simulink model "sampleModel1662"  (R2023a)
settings: Solver=VariableStepAuto  StartTime=0.0  StopTime=10.0  RelTol=1e-3
libraries: hdlsllib x5, simulink x2
settings Model: Creator=user1  LastModifiedBy=user1

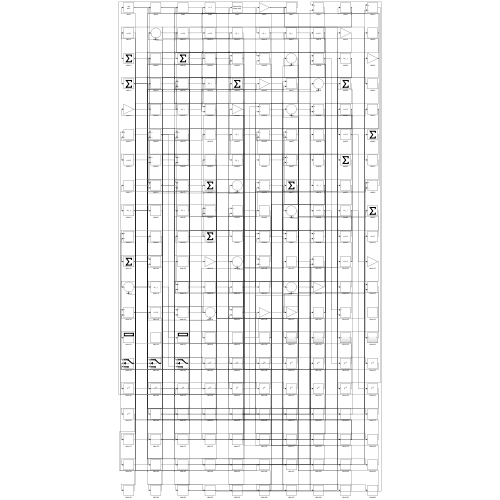
[thumbnail: Simulink's stored preview of the top-level diagram]
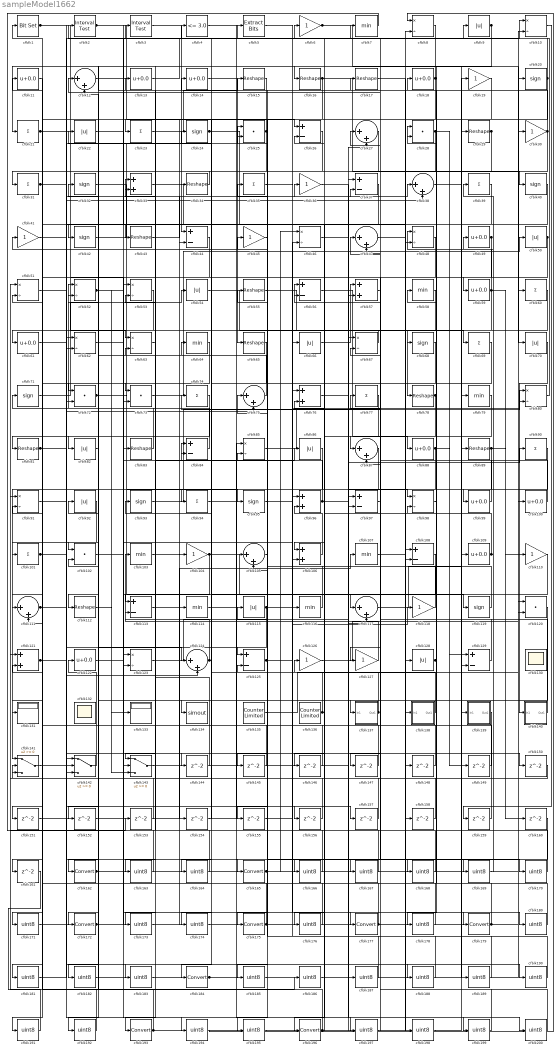
== system sampleModel1662 ==
  cfblk1 : simulink/Logic and Bit Operations/Bit Set  iBit=0
      settings: LibrarySourceBlock=|
      | hdlsllib/Logic and Bit
      | Operations/Bit Set
  cfblk{8,10,46,48,51..53,62..63,67,80,85,91,98,123} (15 alike) : Product  Inputs=*/  RndMeth=Zero  SaturateOnIntegerOverflow=on
  cfblk{11,13..14,18,49,59,61,88,99..100,109,122} (12 alike) : Bias  Bias=0.0  SaturateOnIntegerOverflow=off
  cfblk{21,23,31,35,39,60,69,74,77,90,94,101} (12 alike) : Sum  Inputs=+
  cfblk{25,28,72..73,102,120} (6 alike) : DotProduct  OutDataTypeStr=Inherit: Inherit via internal rule
  cfblk{7,58,64,79,103,107,114,116} (8 alike) : MinMax
  cfblk{6,19,30,36,41,45,104,110,118,126..127} (11 alike) : Gain
  cfblk{12,27,38,47,75,87,105,111,117,124} (10 alike) : Sum  Inputs=|++
  cfblk{33,57,76,96,106,121} (6 alike) : Sum
  cfblk{26,37,44,56,84,97,108,113,125,129} (10 alike) : Sum  Inputs=+-
  cfblk{15..17,29,34,43,55,65,78,81,83,89,112} (13 alike) : Reshape
  cfblk{9,22,50,54,66,70,82,86,92,115,128} (11 alike) : Abs  SaturateOnIntegerOverflow=off
  cfblk{20,24,32,40,42,68,71,93,95,119} (10 alike) : Signum
  cfblk130 : Scope
      settings: Floating=on
  cfblk131 : Display
  cfblk132 : Scope
      settings: Floating=on
  cfblk133 : Display
  cfblk134 : ToWorkspace  VariableName=simout  SaveFormat=Timeseries  SampleTime=-1
  cfblk135 : hdlsllib/Sources/Counter Limited  uplimit=7  tsamp=-1
  cfblk136 : hdlsllib/Sources/Counter Limited  uplimit=7  tsamp=-1
  cfblk137 : Subsystem
      settings: LibrarySourceBlock=|
      | hdlsllib/Ports &
      | Subsystems/Subsystem
  cfblk138 : Subsystem
      settings: LibrarySourceBlock=|
      | hdlsllib/Ports &
      | Subsystems/Subsystem
  cfblk139 : Subsystem
      settings: LibrarySourceBlock=|
      | hdlsllib/Ports &
      | Subsystems/Subsystem
  cfblk140 : Subsystem
      settings: LibrarySourceBlock=|
      | hdlsllib/Ports &
      | Subsystems/Subsystem
  cfblk141 : Switch  SaturateOnIntegerOverflow=off  InputSameDT=off
  cfblk142 : Switch  SaturateOnIntegerOverflow=off  InputSameDT=off
  cfblk143 : Switch  SaturateOnIntegerOverflow=off  InputSameDT=off
  cfblk{144..161} (18 alike) : Delay  SampleTime=1
  cfblk{162,165,172,175,177,179,184,193,196} (9 alike) : DataTypeConversion  SaturateOnIntegerOverflow=off  RndMeth=Floor
  cfblk{163..164,166..171,173..174,176,178,180..183,185..192,194..195,197..200} (30 alike) : DataTypeConversion  OutDataTypeStr=uint8  SaturateOnIntegerOverflow=off  RndMeth=Floor
  cfblk2 : hdlsllib/Logic and Bit Operations/Interval Test  IntervalClosedRight=on  uplimit=0.5  IntervalClosedLeft=on  lowlimit=-0.5  OutDataTypeStr=boolean
  cfblk3 : hdlsllib/Logic and Bit Operations/Interval Test  IntervalClosedRight=on  uplimit=0.5  IntervalClosedLeft=on  lowlimit=-0.5  OutDataTypeStr=boolean
  cfblk4 : hdlsllib/Logic and Bit Operations/Compare To Constant  relop=<=  const=3.0  OutDataTypeStr=boolean
  cfblk5 : simulink/Logic and Bit Operations/Extract Bits  bitsToExtract=Upper half  numBits=8  bitIdxRange=[0 7]  outScalingMode=Preserve fixed-point scaling
      settings: LibrarySourceBlock=|
      | hdlsllib/Logic and Bit
      | Operations/Extract Bits
  wires:
  cfblk31/1 -> cfblk10/1, cfblk43/1, cfblk166/1
  cfblk70/1 -> cfblk140/1(In1)
  cfblk80/1 -> cfblk9/1
  cfblk108/1 -> cfblk184/1
  cfblk50/1 -> cfblk101/1, cfblk155/1
  cfblk45/1 -> cfblk175/1
  cfblk56/1 -> cfblk88/1
  cfblk49/1 -> cfblk59/1, cfblk173/1
  cfblk93/1 -> cfblk80/1
  cfblk32/1 -> cfblk117/1
  cfblk30/1 -> cfblk21/1, cfblk72/2
  cfblk126/1 -> cfblk30/1
  cfblk14/1 -> cfblk65/1
  cfblk123/1 -> cfblk90/1
  cfblk51/1 -> cfblk165/1
  cfblk115/1 -> cfblk66/1, cfblk192/1
  cfblk90/1 -> cfblk106/1
  cfblk23/1 -> cfblk15/1
  cfblk127/1 -> cfblk103/1
  cfblk68/1 -> cfblk134/1
  cfblk121/1 -> cfblk75/2, cfblk183/1
  cfblk67/1 -> cfblk61/1
  cfblk1/1 -> cfblk63/1, cfblk124/2
  cfblk138/1(Out1) -> cfblk84/1
  cfblk73/1 -> cfblk50/1
  cfblk87/1 -> cfblk141/1
  cfblk72/1 -> cfblk95/1, cfblk7/1
  cfblk34/1 -> cfblk31/1
  cfblk104/1 -> cfblk119/1, cfblk143/2
  cfblk59/1 -> cfblk87/1, cfblk48/1, cfblk110/1
  cfblk5/1 -> cfblk116/1
  cfblk71/1 -> cfblk54/1
  cfblk95/1 -> cfblk80/2
  cfblk58/1 -> cfblk78/1
  cfblk44/1 -> cfblk102/1
  cfblk98/1 -> cfblk58/1
  cfblk83/1 -> cfblk52/1
  cfblk36/1 -> cfblk97/1
  cfblk18/1 -> cfblk16/1, cfblk73/1, cfblk42/1
  cfblk112/1 -> cfblk133/1
  cfblk28/1 -> cfblk149/1, cfblk163/1
  cfblk97/1 -> cfblk127/1
  cfblk66/1 -> cfblk57/1
  cfblk117/1 -> cfblk89/1
  cfblk25/1 -> cfblk23/1, cfblk72/1
  cfblk16/1 -> cfblk40/1, cfblk142/3
  cfblk128/1 -> cfblk28/1, cfblk98/2
  cfblk143/1 -> cfblk67/1
  cfblk100/1 -> cfblk56/1
  cfblk65/1 -> cfblk94/1
  cfblk53/1 -> cfblk162/1
  cfblk81/1 -> cfblk37/2, cfblk38/1, cfblk169/1
  cfblk139/1(Out1) -> cfblk141/2
  cfblk142/1 -> cfblk122/1
  cfblk74/1 -> cfblk131/1
  cfblk12/1 -> cfblk104/1
  cfblk77/1 -> cfblk196/1
  cfblk21/1 -> cfblk83/1, cfblk111/1
  cfblk55/1 -> cfblk69/1
  cfblk42/1 -> cfblk25/1
  cfblk136/1 -> cfblk22/1, cfblk6/1
  cfblk3/1 -> cfblk44/1
  cfblk89/1 -> cfblk99/1, cfblk113/1, cfblk160/1
  cfblk119/1 -> cfblk41/1
  cfblk9/1 -> cfblk68/1, cfblk152/1
  cfblk20/1 -> cfblk2/1, cfblk34/1
  cfblk85/1 -> cfblk19/1
  cfblk2/1 -> cfblk26/1, cfblk48/2
  cfblk135/1 -> cfblk20/1
  cfblk118/1 -> cfblk27/1
  cfblk54/1 -> cfblk97/2
  cfblk84/1 -> cfblk71/1
  cfblk82/1 -> cfblk112/1
  cfblk96/1 -> cfblk13/1, cfblk200/1
  cfblk137/1(Out1) -> cfblk93/1, cfblk64/1
  cfblk40/1 -> cfblk81/1
  cfblk43/1 -> cfblk36/1
  cfblk116/1 -> cfblk14/1
  cfblk22/1 -> cfblk44/2
  cfblk52/1 -> cfblk123/2, cfblk106/2, cfblk143/3
  cfblk26/1 -> cfblk82/1
  cfblk109/1 -> cfblk49/1, cfblk26/2
  cfblk99/1 -> cfblk12/1
  cfblk33/1 -> cfblk105/1
  cfblk57/1 -> cfblk17/1
  cfblk101/1 -> cfblk124/1, cfblk156/1
  cfblk129/1 -> cfblk3/1
  cfblk6/1 -> cfblk70/1, cfblk139/1(In1)
  cfblk63/1 -> cfblk33/1
  cfblk111/1 -> cfblk38/2, cfblk150/1
  cfblk120/1 -> cfblk172/1
  cfblk13/1 -> cfblk5/1
  cfblk141/1 -> cfblk24/1
  cfblk29/1 -> cfblk125/1, cfblk129/2
  cfblk62/1 -> cfblk179/1
  cfblk102/1 -> cfblk86/1
  cfblk24/1 -> cfblk57/2, cfblk174/1
  cfblk106/1 -> cfblk96/2
  cfblk125/1 -> cfblk55/1, cfblk118/1
  cfblk124/1 -> cfblk4/1, cfblk113/2
  cfblk88/1 -> cfblk143/1, cfblk129/1
  cfblk105/1 -> cfblk85/2
  cfblk8/1 -> cfblk193/1
  cfblk140/1(Out1) -> cfblk74/1
  cfblk79/1 -> cfblk137/1(In1)
  cfblk113/1 -> cfblk107/1
  cfblk46/1 -> cfblk98/1
  cfblk78/1 -> cfblk146/1, cfblk147/1
  cfblk35/1 -> cfblk177/1
  cfblk75/1 -> cfblk32/1
  cfblk61/1 -> cfblk144/1
  cfblk144/1 -> cfblk63/2
  cfblk86/1 -> cfblk145/1
  cfblk145/1 -> cfblk1/1
  cfblk146/1 -> cfblk33/2
  cfblk147/1 -> cfblk105/2
  cfblk148/1 -> cfblk12/2
  cfblk149/1 -> cfblk87/2
  cfblk150/1 -> cfblk141/3
  cfblk15/1 -> cfblk151/1
  cfblk151/1 -> cfblk85/1
  cfblk7/1 -> cfblk153/1
  cfblk153/1 -> cfblk121/1
  cfblk103/1 -> cfblk154/1
  cfblk154/1 -> cfblk84/2
  cfblk155/1 -> cfblk96/1
  cfblk156/1 -> cfblk75/1
  cfblk4/1 -> cfblk157/1
  cfblk157/1 -> cfblk142/1
  cfblk107/1 -> cfblk158/1
  cfblk158/1 -> cfblk123/1
  cfblk10/1 -> cfblk159/1
  cfblk159/1 -> cfblk125/2
  cfblk64/1 -> cfblk161/1
  cfblk162/1 -> cfblk148/1, cfblk46/2
  cfblk163/1 -> cfblk53/1
  cfblk110/1 -> cfblk164/1
  cfblk164/1 -> cfblk53/2
  cfblk165/1 -> cfblk128/1, cfblk10/2, cfblk46/1
  cfblk166/1 -> cfblk51/1
  cfblk48/1 -> cfblk167/1
  cfblk167/1 -> cfblk51/2
  cfblk39/1 -> cfblk168/1
  cfblk168/1 -> cfblk102/2
  cfblk169/1 -> cfblk39/1
  cfblk114/1 -> cfblk170/1
  cfblk170/1 -> cfblk18/1
  cfblk11/1 -> cfblk171/1
  cfblk171/1 -> cfblk114/1
  cfblk172/1 -> cfblk73/2, cfblk138/1(In1)
  cfblk173/1 -> cfblk120/1
  cfblk174/1 -> cfblk120/2
  cfblk175/1 -> cfblk115/1, cfblk117/2, cfblk92/1
  cfblk37/1 -> cfblk176/1
  cfblk176/1 -> cfblk45/1
  cfblk177/1 -> cfblk11/1, cfblk142/2
  cfblk69/1 -> cfblk178/1
  cfblk178/1 -> cfblk35/1
  cfblk179/1 -> cfblk111/2, cfblk28/2, cfblk67/2
  cfblk17/1 -> cfblk180/1
  cfblk180/1 -> cfblk62/1
  cfblk27/1 -> cfblk181/1
  cfblk181/1 -> cfblk62/2
  cfblk60/1 -> cfblk182/1
  cfblk182/1 -> cfblk100/1
  cfblk183/1 -> cfblk60/1
  cfblk184/1 -> cfblk37/1, cfblk29/1
  cfblk19/1 -> cfblk185/1
  cfblk185/1 -> cfblk108/1
  cfblk161/1 -> cfblk186/1
  cfblk186/1 -> cfblk108/2
  cfblk76/1 -> cfblk187/1
  cfblk187/1 -> cfblk25/2
  cfblk152/1 -> cfblk188/1
  cfblk188/1 -> cfblk76/1
  cfblk38/1 -> cfblk189/1
  cfblk189/1 -> cfblk76/2
  cfblk91/1 -> cfblk190/1
  cfblk190/1 -> cfblk56/2
  cfblk92/1 -> cfblk191/1
  cfblk191/1 -> cfblk91/1
  cfblk192/1 -> cfblk91/2
  cfblk193/1 -> cfblk79/1, cfblk27/2, cfblk121/2
  cfblk122/1 -> cfblk194/1
  cfblk194/1 -> cfblk8/1
  cfblk160/1 -> cfblk195/1
  cfblk195/1 -> cfblk8/2
  cfblk196/1 -> cfblk52/2, cfblk126/1
  cfblk41/1 -> cfblk197/1
  cfblk197/1 -> cfblk77/1
  cfblk47/1 -> cfblk198/1
  cfblk198/1 -> cfblk109/1
  cfblk94/1 -> cfblk199/1
  cfblk199/1 -> cfblk47/1
  cfblk200/1 -> cfblk47/2

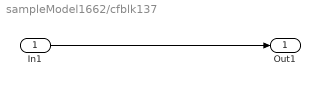
== system sampleModel1662/cfblk137 ==
  In1 : Inport
  Out1 : Outport
  wires:
  In1/1 -> Out1/1

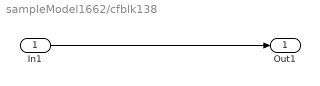
== system sampleModel1662/cfblk138 ==
  In1 : Inport
  Out1 : Outport
  wires:
  In1/1 -> Out1/1

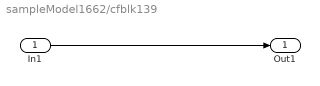
== system sampleModel1662/cfblk139 ==
  In1 : Inport
  Out1 : Outport
  wires:
  In1/1 -> Out1/1

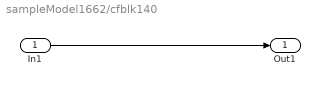
== system sampleModel1662/cfblk140 ==
  In1 : Inport
  Out1 : Outport
  wires:
  In1/1 -> Out1/1
